simulink model "rv32i"  (R2018a)
settings: Solver=VariableStepAuto  StartTime=0.0  StopTime=10.0  RelTol=1e-3
settings Model: Creator=Hagi  LastModifiedBy=Hagi

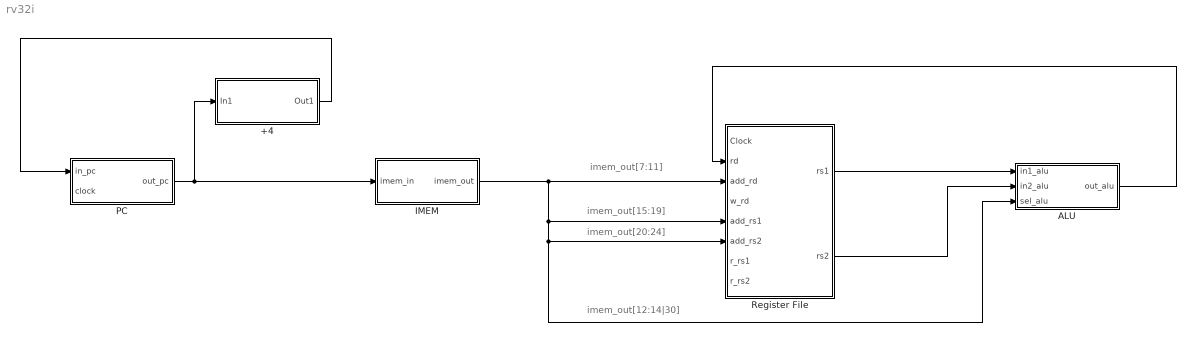
== system rv32i ==
  note: imem_out[7:11]
  note: imem_out[15:19]
  note: imem_out[20:24]
  note: imem_out[12:14|30]
  +4 : Subsystem
  ALU : Subsystem
  IMEM : Subsystem
  PC : Subsystem
  Register File : Subsystem
  wires:
  Register File/2(rs2) -> ALU/2(in2_alu)
  Register File/1(rs1) -> ALU/1(in1_alu)
  ALU/1(out_alu) -> Register File/2(rd)
  IMEM/1(imem_out) -> Register File/6(add_rs2), ALU/3(sel_alu), Register File/5(add_rs1), Register File/3(add_rd)
  PC/1(out_pc) -> IMEM/1(imem_in), +4/1(In1)
  +4/1(Out1) -> PC/1(in_pc)

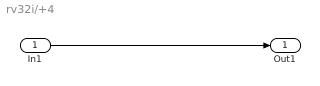
== system rv32i/+4 ==
  In1 : Inport
  Out1 : Outport
  wires:
  In1/1 -> Out1/1

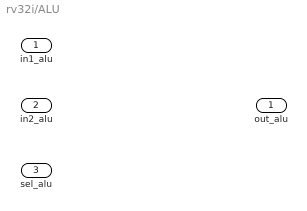
== system rv32i/ALU ==
  in1_alu : Inport
  in2_alu : Inport  Port=2
  sel_alu : Inport  Port=3
  out_alu : Outport

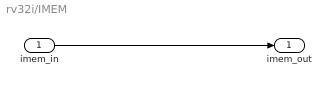
== system rv32i/IMEM ==
  imem_in : Inport
  imem_out : Outport
  wires:
  imem_in/1 -> imem_out/1

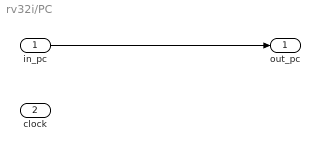
== system rv32i/PC ==
  in_pc : Inport
  clock : Inport  Port=2
  out_pc : Outport
  wires:
  in_pc/1 -> out_pc/1

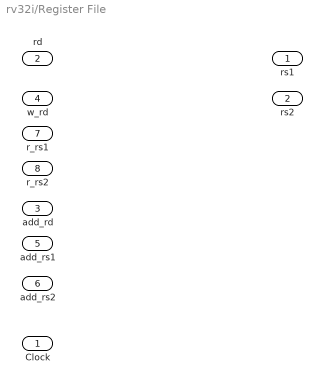
== system rv32i/Register File ==
  Clock : Inport
  rd : Inport  Port=2
  add_rd : Inport  Port=3
  w_rd : Inport  Port=4
  add_rs1 : Inport  Port=5
  add_rs2 : Inport  Port=6
  r_rs1 : Inport  Port=7
  r_rs2 : Inport  Port=8
  rs1 : Outport
  rs2 : Outport  Port=2
